simulink model "STEMMS_VOLTAGE_COMMENTED_V2"  (R2019b)
settings: Solver=FixedStepAuto  StartTime=0.0  StopTime=inf  RelTol=1e-3
libraries: vexarmcortexlib x26, vexcommonlib x7
settings Model: ExtModeTrigDuration=25  Creator=nicoa  LastModifiedBy=nicoa
settings OptimizationCC: EnhancedBackFolding=on  PassReuseOutputArgsAs=Individual arguments  ZeroExternalMemoryAtStartup=off  ZeroInternalMemoryAtStartup=off  MaxStackSize=64  OptimizeBlockOrder=speed  DifferentSizesBufferReuse=on  OptimizationCustomize=off  EfficientTunableParamExpr=on
settings DebuggingCC: ParameterTunabilityLossMsg=error
settings HardwareCC: ProdBitPerPointer=32  ProdBitPerSizeT=32  ProdBitPerPtrDiffT=32  ProdLargestAtomicInteger=Long  ProdLargestAtomicFloat=Double  ProdWordSize=32  ProdHWDeviceType=ARM Compatible->ARM Cortex
settings SFSimCC: MATLABDynamicMemAlloc=off
settings RTWCC: SystemTargetFile=ert.tlc  HardwareBoard=ARM Cortex-based VEX Microcontroller  TLCOptions="-aInlineSetEventsForThisBaseRateFcn=TLC_FALSE -aSuppressMultiTaskScheduler=TLC_FALSE  -aRateBasedStepFcn=0"  TemplateMakefile=ert_default_tmf  GenerateReport=on  Toolchain=GNU Tools for VEX ARM Cortex  IncludeHyperlinkInReport=on  LaunchReport=on  GenerateTraceInfo=on  GenerateTraceReport=on  GenerateTraceReportSl=on  GenerateTraceReportSf=on  GenerateTraceReportEml=on
settings CodeAppCC: ForceParamTrailComments=on  IgnoreCustomStorageClasses=off  OperatorAnnotations=on  SimulinkDataObjDesc=on  SFDataObjDesc=on  InsertBlockDesc=on

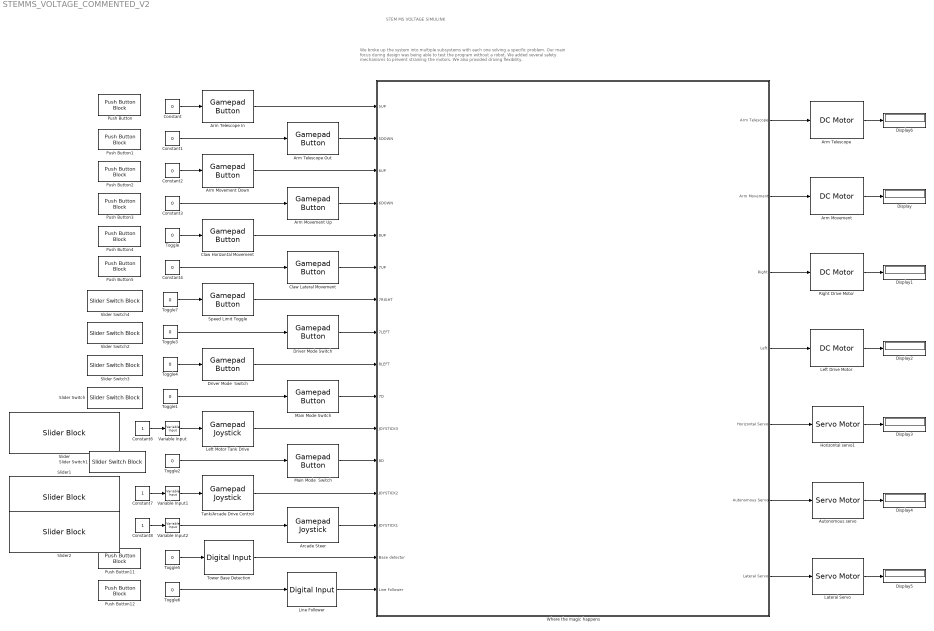
== system STEMMS_VOLTAGE_COMMENTED_V2 ==
  note: We broke up the system into multiple subsystems with each one solving a specific problem. Our main focus during
      | design was being able to test the program without a robot. We added several safety mechanisms to prevent straining
      |  the motors. We also provided driving flexibility.
  note: STEM MS VOLTAGE SIMULINK
  "Arcade Steer " : vexarmcortexlib/Gamepad/Gamepad Joystick  joystick=1  chan=1  SimulationIn=on  SampleTime=0.02
      settings: SourceProductName=Simulink Coder Support Package for ARM Cortex-based VEX Microcontroller  SourceProductBaseCode=EC_VEX_MICRO
  Arm Movement : vexarmcortexlib/Actuators/DC Motor  motor=6  scaleFactor=1/13.5  SimulationOut=on
      settings: SourceProductName=Simulink Coder Support Package for ARM Cortex-based VEX Microcontroller  SourceProductBaseCode=EC_VEX_MICRO
  Arm Movement Down : vexarmcortexlib/Gamepad/Gamepad Button  joystick=1  chan=6  button56=Down  button78=Down  SimulationIn=on  SampleTime=0.02
      settings: SourceProductName=Simulink Coder Support Package for ARM Cortex-based VEX Microcontroller  SourceProductBaseCode=EC_VEX_MICRO
  Arm Movement Up : vexarmcortexlib/Gamepad/Gamepad Button  joystick=1  chan=6  button56=Up  button78=Down  SimulationIn=on  SampleTime=0.02
      settings: SourceProductName=Simulink Coder Support Package for ARM Cortex-based VEX Microcontroller  SourceProductBaseCode=EC_VEX_MICRO
  Arm Telescope : vexarmcortexlib/Actuators/DC Motor  motor=2  scaleFactor=1/13.5  SimulationOut=on
      settings: SourceProductName=Simulink Coder Support Package for ARM Cortex-based VEX Microcontroller  SourceProductBaseCode=EC_VEX_MICRO
  Arm Telescope In : vexarmcortexlib/Gamepad/Gamepad Button  joystick=1  chan=5  button56=Down  button78=Down  SimulationIn=on  SampleTime=0.02
      settings: SourceProductName=Simulink Coder Support Package for ARM Cortex-based VEX Microcontroller  SourceProductBaseCode=EC_VEX_MICRO
  Arm Telescope Out : vexarmcortexlib/Gamepad/Gamepad Button  joystick=1  chan=5  button56=Up  button78=Down  SimulationIn=on  SampleTime=0.02
      settings: SourceProductName=Simulink Coder Support Package for ARM Cortex-based VEX Microcontroller  SourceProductBaseCode=EC_VEX_MICRO
  Autonomous servo : vexarmcortexlib/Actuators/Servo Motor  motor=5  scaleFactor=60/127  SimulationOut=on
      settings: SourceProductName=Simulink Coder Support Package for ARM Cortex-based VEX Microcontroller  SourceProductBaseCode=EC_VEX_MICRO
  Claw Horizontal Movement : vexarmcortexlib/Gamepad/Gamepad Button  joystick=1  chan=8  button56=Up  button78=Up  SimulationIn=on  SampleTime=0.02
      settings: SourceProductName=Simulink Coder Support Package for ARM Cortex-based VEX Microcontroller  SourceProductBaseCode=EC_VEX_MICRO
  Claw Lateral Movement : vexarmcortexlib/Gamepad/Gamepad Button  joystick=1  chan=7  button56=Up  button78=Up  SimulationIn=on  SampleTime=0.02
      settings: SourceProductName=Simulink Coder Support Package for ARM Cortex-based VEX Microcontroller  SourceProductBaseCode=EC_VEX_MICRO
  Constant{,1..4} (5 alike) : Constant  Value=0
  Constant6 : Constant
  Constant7 : Constant
  Constant8 : Constant
  Display{,1..6} (7 alike) : Display
  Driver Mode  Switch : vexarmcortexlib/Gamepad/Gamepad Button  joystick=1  chan=8  button56=Up  button78=Left  SimulationIn=on  SampleTime=0.02
      settings: SourceProductName=Simulink Coder Support Package for ARM Cortex-based VEX Microcontroller  SourceProductBaseCode=EC_VEX_MICRO
  Driver Mode Switch : vexarmcortexlib/Gamepad/Gamepad Button  joystick=1  chan=7  button56=Up  button78=Left  SimulationIn=on  SampleTime=0.02
      settings: SourceProductName=Simulink Coder Support Package for ARM Cortex-based VEX Microcontroller  SourceProductBaseCode=EC_VEX_MICRO
  Horizontal servo1 : vexarmcortexlib/Actuators/Servo Motor  motor=7  scaleFactor=60/127  SimulationOut=on
      settings: SourceProductName=Simulink Coder Support Package for ARM Cortex-based VEX Microcontroller  SourceProductBaseCode=EC_VEX_MICRO
  Lateral Servo : vexarmcortexlib/Actuators/Servo Motor  motor=3  scaleFactor=60/127  SimulationOut=on
      settings: SourceProductName=Simulink Coder Support Package for ARM Cortex-based VEX Microcontroller  SourceProductBaseCode=EC_VEX_MICRO
  "Left Drive Motor " : vexarmcortexlib/Actuators/DC Motor  motor=9  scaleFactor=1/13.5  SimulationOut=on
      settings: SourceProductName=Simulink Coder Support Package for ARM Cortex-based VEX Microcontroller  SourceProductBaseCode=EC_VEX_MICRO
  Left Motor Tank Drive : vexarmcortexlib/Gamepad/Gamepad Joystick  joystick=1  chan=3  SimulationIn=on  SampleTime=0.02
      settings: SourceProductName=Simulink Coder Support Package for ARM Cortex-based VEX Microcontroller  SourceProductBaseCode=EC_VEX_MICRO
  Line Follower : vexarmcortexlib/Sensors/Digital Input  inChan=1  SimulationIn=on  SampleTime=0.2
      settings: SourceProductName=Simulink Coder Support Package for ARM Cortex-based VEX Microcontroller  SourceProductBaseCode=EC_VEX_MICRO
  Main Mode  Switch : vexarmcortexlib/Gamepad/Gamepad Button  joystick=1  chan=8  button56=Up  button78=Down  SimulationIn=on  SampleTime=0.02
      settings: SourceProductName=Simulink Coder Support Package for ARM Cortex-based VEX Microcontroller  SourceProductBaseCode=EC_VEX_MICRO
  Main Mode Switch : vexarmcortexlib/Gamepad/Gamepad Button  joystick=1  chan=7  button56=Up  button78=Down  SimulationIn=on  SampleTime=0.02
      settings: SourceProductName=Simulink Coder Support Package for ARM Cortex-based VEX Microcontroller  SourceProductBaseCode=EC_VEX_MICRO
  Push Button{,1..5,11..12} (8 alike) : PushButtonBlock
  Right Drive Motor : vexarmcortexlib/Actuators/DC Motor  motor=4  scaleFactor=1/13.5  SimulationOut=on
      settings: SourceProductName=Simulink Coder Support Package for ARM Cortex-based VEX Microcontroller  SourceProductBaseCode=EC_VEX_MICRO
  Slider : SliderBlock  LabelPosition=Hide  ScaleMin=-127  ScaleMax=127
  Slider Switch{,1..4} (5 alike) : SliderSwitchBlock  LabelPosition=Hide
      settings: Values={{'Off', 'On'}, [0 1]}
  Slider1 : SliderBlock  LabelPosition=Hide  ScaleMin=-127  ScaleMax=127
  Slider2 : SliderBlock  LabelPosition=Hide  ScaleMin=-127  ScaleMax=127
  Speed Limit Toggle : vexarmcortexlib/Gamepad/Gamepad Button  joystick=1  chan=7  button56=Up  button78=Right  SimulationIn=on  SampleTime=0.02
      settings: SourceProductName=Simulink Coder Support Package for ARM Cortex-based VEX Microcontroller  SourceProductBaseCode=EC_VEX_MICRO
  Tank/Arcade Drive Control : vexarmcortexlib/Gamepad/Gamepad Joystick  joystick=1  chan=2  SimulationIn=on  SampleTime=0.02
      settings: SourceProductName=Simulink Coder Support Package for ARM Cortex-based VEX Microcontroller  SourceProductBaseCode=EC_VEX_MICRO
  Toggle{,1..7} (8 alike) : Constant  Value=0
      settings: OpenFcn=|
      | if strcmp('0',get_param(gcb, 'Value'))                        set_param(gcb, 'Value', '1');
      | else
      |             set_param(gcb, 'Value', '0');
      | end
  Tower Base Detection : vexarmcortexlib/Sensors/Digital Input  inChan=11  SimulationIn=on  SampleTime=0.2
      settings: SourceProductName=Simulink Coder Support Package for ARM Cortex-based VEX Microcontroller  SourceProductBaseCode=EC_VEX_MICRO
  Variable Input : vexarmcortexlib/Utilities/Variable Input  low=-127  gain=94.76544331395348  high=127
      settings: SourceProductName=Simulink Coder Support Package for ARM Cortex-based VEX Microcontroller  SourceProductBaseCode=EC_VEX_MICRO
  Variable Input1 : vexarmcortexlib/Utilities/Variable Input  low=-127  gain=-87  high=127
      settings: SourceProductName=Simulink Coder Support Package for ARM Cortex-based VEX Microcontroller  SourceProductBaseCode=EC_VEX_MICRO
  Variable Input2 : vexarmcortexlib/Utilities/Variable Input  low=-127  gain=56.37009447674421  high=127
      settings: SourceProductName=Simulink Coder Support Package for ARM Cortex-based VEX Microcontroller  SourceProductBaseCode=EC_VEX_MICRO
  Where the magic happens : Subsystem
  wires:
  Main Mode  Switch/1 -> Where the magic happens/12(8D)
  Main Mode Switch/1 -> Where the magic happens/10(7D)
  Where the magic happens/4(Left) -> "Left Drive Motor "/1
  Where the magic happens/6(Autonomous Servo) -> Autonomous servo/1
  Tower Base Detection/1 -> Where the magic happens/15(Base detector)
  Line Follower/1 -> Where the magic happens/16(Line Follower)
  Driver Mode  Switch/1 -> Where the magic happens/9(8LEFT)
  Driver Mode Switch/1 -> Where the magic happens/8(7LEFT)
  Speed Limit Toggle/1 -> Where the magic happens/7(7RIGHT)
  Tank/Arcade Drive Control/1 -> Where the magic happens/13(JOYSTICK2)
  Left Motor Tank Drive/1 -> Where the magic happens/11(JOYSTICK3)
  "Arcade Steer "/1 -> Where the magic happens/14(JOYSTICK1)
  Where the magic happens/3(Right) -> Right Drive Motor/1
  Where the magic happens/7(Lateral Servo) -> Lateral Servo/1
  Where the magic happens/5(Horizontal Servo) -> Horizontal servo1/1
  Claw Lateral Movement/1 -> Where the magic happens/6(7UP)
  Claw Horizontal Movement/1 -> Where the magic happens/5(8UP)
  Where the magic happens/2(Arm Movement) -> Arm Movement/1
  Arm Movement Up/1 -> Where the magic happens/4(6DOWN)
  Arm Movement Down/1 -> Where the magic happens/3(6UP)
  Where the magic happens/1(Arm Telescope) -> Arm Telescope/1
  Arm Telescope Out/1 -> Where the magic happens/2(5DOWN)
  Arm Telescope In/1 -> Where the magic happens/1(5UP)
  Arm Movement/1 -> Display/1
  Right Drive Motor/1 -> Display1/1
  "Left Drive Motor "/1 -> Display2/1
  Horizontal servo1/1 -> Display3/1
  Autonomous servo/1 -> Display4/1
  Lateral Servo/1 -> Display5/1
  Arm Telescope/1 -> Display6/1
  Constant/1 -> Arm Telescope In/1
  Constant1/1 -> Arm Telescope Out/1
  Constant2/1 -> Arm Movement Down/1
  Constant3/1 -> Arm Movement Up/1
  Toggle/1 -> Claw Horizontal Movement/1
  Constant4/1 -> Claw Lateral Movement/1
  Toggle7/1 -> Speed Limit Toggle/1
  Toggle4/1 -> Driver Mode  Switch/1
  Toggle1/1 -> Main Mode Switch/1
  Constant6/1 -> Variable Input/1
  Variable Input/1 -> Left Motor Tank Drive/1
  Variable Input1/1 -> Tank/Arcade Drive Control/1
  Constant7/1 -> Variable Input1/1
  Variable Input2/1 -> "Arcade Steer "/1
  Constant8/1 -> Variable Input2/1
  Toggle2/1 -> Main Mode  Switch/1
  Toggle5/1 -> Tower Base Detection/1
  Toggle6/1 -> Line Follower/1
  Toggle3/1 -> Driver Mode Switch/1

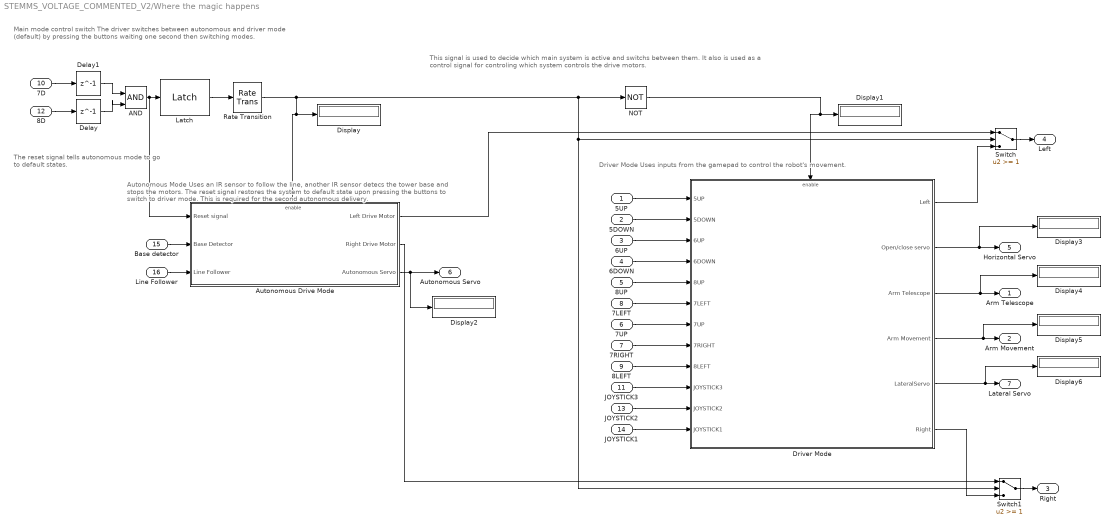
== system STEMMS_VOLTAGE_COMMENTED_V2/Where the magic happens ==
  note: Driver Mode
      | Uses inputs from the gamepad to control the robot's movement.
  note: This signal is used to decide which main system is active and switchs between them.
      | It also is used as a control signal for controling which system controls the drive motors.
  note: The reset signal tells autonomous
      | mode to go to default states.
  note: Autonomous Mode
      | Uses an IR sensor to follow the line, another IR sensor detecs the
      | tower base and stops the motors. The reset signal restores the system
      | to default state upon pressing the buttons to switch to driver mode. This
      | is required for the second autonomous delivery.
  note: Main mode control switch
      | The driver switches between autonomous and driver mode (default) by
      | pressing the buttons waiting one second then switching modes.
  5UP : Inport
  5DOWN : Inport  Port=2
  6UP : Inport  Port=3
  6DOWN : Inport  Port=4
  8UP : Inport  Port=5
  7UP : Inport  Port=6
  7RIGHT : Inport  Port=7
  7LEFT : Inport  Port=8
  8LEFT : Inport  Port=9
  7D : Inport  Port=10
  JOYSTICK3 : Inport  Port=11
  8D : Inport  Port=12
  JOYSTICK2 : Inport  Port=13
  JOYSTICK1 : Inport  Port=14
  Base detector : Inport  Port=15
  Line Follower : Inport  Port=16
  "AND " : Logic  IconShape=distinctive  AllPortsSameDT=off  OutDataTypeStr=boolean
  Autonomous Drive Mode : Subsystem
  Delay : Delay  DelayLength=1  InitialCondition=0  SampleTime=1
  Delay1 : Delay  DelayLength=1  InitialCondition=0  SampleTime=1
  Display{,1..6} (7 alike) : Display
  Driver Mode : Subsystem  TreatAsAtomicUnit=on
  Latch : vexcommonlib/Latch  output0=off  BlockPlatform=vexarmcortex
      settings: SourceProductName=Simulink Coder Support Package for ARM Cortex-based VEX Microcontroller  SourceProductBaseCode=EC_VEX_MICRO
  NOT : Logic  Operator=NOT  IconShape=distinctive  AllPortsSameDT=off  OutDataTypeStr=boolean
  Rate Transition : RateTransition
  Switch : Switch  Threshold=1
  Switch1 : Switch  Threshold=1
  Arm Telescope : Outport
  Arm Movement : Outport  Port=2
  Right : Outport  Port=3
  Left : Outport  Port=4
  Horizontal Servo : Outport  Port=5
  Autonomous Servo : Outport  Port=6
  Lateral Servo : Outport  Port=7
  wires:
  "AND "/1 -> Autonomous Drive Mode/1(Reset signal), Latch/1
  Delay1/1 -> "AND "/1
  Latch/1 -> Rate Transition/1
  7D/1 -> Delay1/1
  Delay/1 -> "AND "/2
  8D/1 -> Delay/1
  Autonomous Drive Mode/3(Autonomous Servo) -> Display2/1, Autonomous Servo/1
  Rate Transition/1 -> Display/1, Autonomous Drive Mode/Enable, NOT/1, Switch1/2, Switch/2
  NOT/1 -> Display1/1, Driver Mode/Enable
  Autonomous Drive Mode/1(Left Drive Motor) -> Switch/1
  Switch/1 -> Left/1
  Autonomous Drive Mode/2(Right Drive Motor) -> Switch1/1
  Switch1/1 -> Right/1
  Line Follower/1 -> Autonomous Drive Mode/3(Line Follower)
  Base detector/1 -> Autonomous Drive Mode/2(Base Detector)
  7RIGHT/1 -> Driver Mode/8(7RIGHT)
  JOYSTICK3/1 -> Driver Mode/10(JOYSTICK3)
  JOYSTICK2/1 -> Driver Mode/11(JOYSTICK2)
  JOYSTICK1/1 -> Driver Mode/12(JOYSTICK1)
  Driver Mode/5(LateralServo) -> Display6/1, Lateral Servo/1
  Driver Mode/2(Open/close servo) -> Display3/1, Horizontal Servo/1
  8UP/1 -> Driver Mode/5(8UP)
  7UP/1 -> Driver Mode/7(7UP)
  Driver Mode/4(Arm Movement) -> Display5/1, Arm Movement/1
  Driver Mode/3(Arm Telescope) -> Display4/1, Arm Telescope/1
  Driver Mode/6(Right) -> Switch1/3
  Driver Mode/1(Left) -> Switch/3
  5DOWN/1 -> Driver Mode/2(5DOWN)
  5UP/1 -> Driver Mode/1(5UP)
  6UP/1 -> Driver Mode/3(6UP)
  6DOWN/1 -> Driver Mode/4(6DOWN)
  7LEFT/1 -> Driver Mode/6(7LEFT)
  8LEFT/1 -> Driver Mode/9(8LEFT)

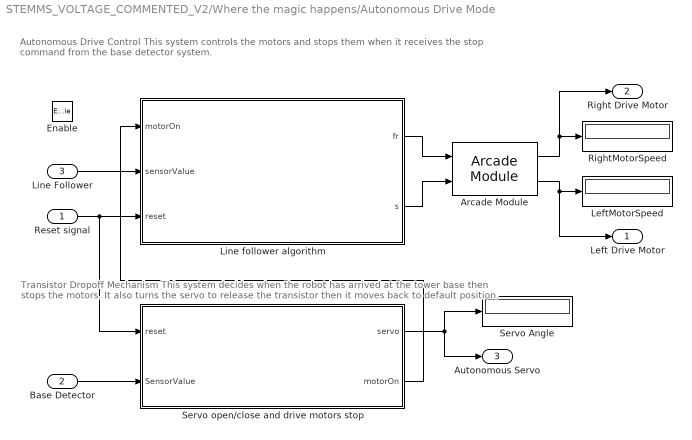
== system STEMMS_VOLTAGE_COMMENTED_V2/Where the magic happens/Autonomous Drive Mode ==
  note: Transistor Dropoff Mechanism
      | This system decides when the robot has arrived at the tower base then stops the motors. It also turns the servo to
      | release the transistor then it moves back to default position.
  note: Autonomous Drive Control
      | This system controls the motors and stops them when it receives the stop command from the base detector system.
  Reset signal : Inport
  Base Detector : Inport  Port=2
  Line Follower : Inport  Port=3
  Enable : EnablePort
  Arcade Module : vexcommonlib/Arcade Module  BlockPlatform=vexarmcortex
      settings: SourceProductName=Simulink Coder Support Package for ARM Cortex-based VEX Microcontroller  SourceProductBaseCode=EC_VEX_MICRO
  LeftMotorSpeed : Display
  Line follower algorithm : Stateflow chart  TreatAsAtomicUnit=on
  RightMotorSpeed : Display
  Servo Angle : Display
  Servo open/close and drive motors stop : Stateflow chart  TreatAsAtomicUnit=on
  Left Drive Motor : Outport
  Right Drive Motor : Outport  Port=2
  Autonomous Servo : Outport  Port=3
  wires:
  Base Detector/1 -> Servo open/close and drive motors stop/2(SensorValue)
  Line Follower/1 -> Line follower algorithm/2(sensorValue)
  Line follower algorithm/2(s) -> Arcade Module/2
  Line follower algorithm/1(fr) -> Arcade Module/1
  Arcade Module/1 -> RightMotorSpeed/1, Right Drive Motor/1
  Arcade Module/2 -> LeftMotorSpeed/1, Left Drive Motor/1
  Servo open/close and drive motors stop/1(servo) -> Autonomous Servo/1, Servo Angle/1
  Servo open/close and drive motors stop/2(motorOn) -> Line follower algorithm/1(motorOn)
  Reset signal/1 -> Servo open/close and drive motors stop/1(reset), Line follower algorithm/3(reset)

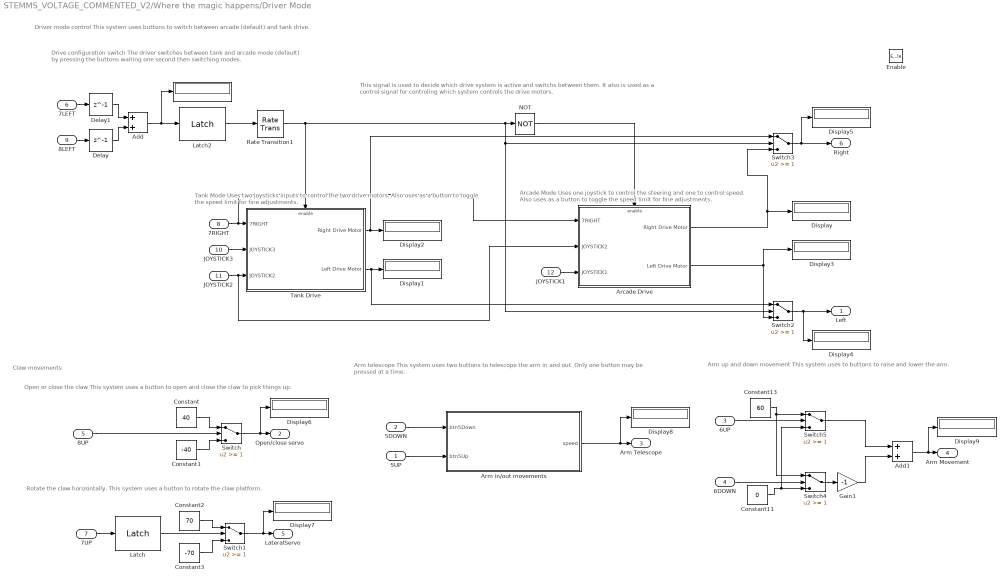
== system STEMMS_VOLTAGE_COMMENTED_V2/Where the magic happens/Driver Mode ==
  note: Rotate the claw horizontally.
      | This system uses a button to rotate the claw platform.
  note: Open or close the claw
      | This system uses a button to open and close the
      | claw to pick things up.
  note: Arcade Mode
      | Uses one joystick to control the steering and one to control
      | speed. Also uses as a button to toggle the speed limit for fine
      | adjustments.
  note: Tank Mode
      | Uses two joysticks inputs to control the two drive motors. Also uses as a button
      | to toggle the speed limit for fine adjustments.
  note: Drive configuration switch
      | The driver switches between tank and arcade mode (default) by
      | pressing the buttons waiting one second then switching modes.
  note: Arm telescope
      | This system uses two buttons to telescope the arm in and out.
      | Only one button may be pressed at a time.
  note: Claw movements
  note: Arm up and down movement
      | This system uses to buttons to raise and lower the arm.
  note: Driver mode control
      | This system uses buttons to switch between arcade (default) and tank drive.
  note: This signal is used to decide which drive system is active and switchs between them.
      | It also is used as a control signal for controling which system controls the drive motors.
  5UP : Inport
  5DOWN : Inport  Port=2
  6UP : Inport  Port=3
  6DOWN : Inport  Port=4
  8UP : Inport  Port=5
  7LEFT : Inport  Port=6
  7UP : Inport  Port=7
  7RIGHT : Inport  Port=8
  8LEFT : Inport  Port=9
  JOYSTICK3 : Inport  Port=10
  JOYSTICK2 : Inport  Port=11
  JOYSTICK1 : Inport  Port=12
  Enable : EnablePort
  " " : Display
  Add : Sum
  Add1 : Sum
  "Arcade Drive " : Subsystem  TreatAsAtomicUnit=on
  Arm in/out movements : Stateflow chart  BlockKeywords=__PRM__SERIALIZED__DATA__:Stateflow Chart,Stateflow Diagram  TreatAsAtomicUnit=on
  Constant : Constant  Value=40
  Constant1 : Constant  Value=-40
  Constant11 : Constant  Value=0
  Constant13 : Constant  Value=60
  Constant2 : Constant  Value=70
  Constant3 : Constant  Value=-70
  Delay : Delay  DelayLength=1  InitialCondition=0  SampleTime=1
  Delay1 : Delay  DelayLength=1  InitialCondition=0  SampleTime=1
  Display{,1..9} (10 alike) : Display
  Gain1 : Gain  Gain=-1
  Latch : vexcommonlib/Latch  output0=off  BlockPlatform=vexarmcortex
      settings: SourceProductName=Simulink Coder Support Package for ARM Cortex-based VEX Microcontroller  SourceProductBaseCode=EC_VEX_MICRO
  Latch2 : vexcommonlib/Latch  output0=off  BlockPlatform=vexarmcortex
      settings: SourceProductName=Simulink Coder Support Package for ARM Cortex-based VEX Microcontroller  SourceProductBaseCode=EC_VEX_MICRO
  NOT : Logic  Operator=NOT  IconShape=distinctive  AllPortsSameDT=off  OutDataTypeStr=boolean
  Rate Transition1 : RateTransition
  Switch{,1..5} (6 alike) : Switch  Threshold=1
  "Tank Drive " : Subsystem  TreatAsAtomicUnit=on
  Left : Outport
  Open/close servo : Outport  Port=2
  Arm Telescope : Outport  Port=3
  Arm Movement : Outport  Port=4
  LateralServo : Outport  Port=5
  Right : Outport  Port=6
  wires:
  Rate Transition1/1 -> NOT/1, Switch2/2, Switch3/2, "Tank Drive "/Enable
  7LEFT/1 -> Delay1/1
  NOT/1 -> "Arcade Drive "/Enable
  Delay1/1 -> Add/1
  Delay/1 -> Add/2
  Latch2/1 -> Rate Transition1/1
  Add/1 -> " "/1, Latch2/1
  8LEFT/1 -> Delay/1
  JOYSTICK3/1 -> "Tank Drive "/2(JOYSTICK3)
  JOYSTICK2/1 -> "Tank Drive "/3(JOYSTICK2), "Arcade Drive "/2(JOYSTICK2)
  JOYSTICK1/1 -> "Arcade Drive "/3(JOYSTICK1)
  Constant/1 -> Switch/1
  7UP/1 -> Latch/1
  Latch/1 -> Switch1/2
  Switch/1 -> Display6/1, Open/close servo/1
  Constant1/1 -> Switch/3
  Switch1/1 -> Display7/1, LateralServo/1
  Constant2/1 -> Switch1/1
  Constant3/1 -> Switch1/3
  Switch4/1 -> Gain1/1
  Constant11/1 -> Switch5/3, Switch4/3
  6DOWN/1 -> Switch4/2
  6UP/1 -> Switch5/2
  Constant13/1 -> Switch5/1, Switch4/1
  Add1/1 -> Display9/1, Arm Movement/1
  5UP/1 -> Arm in/out movements/2(btn5Up)
  Arm in/out movements/1(speed) -> Display8/1, Arm Telescope/1
  5DOWN/1 -> Arm in/out movements/1(btn5Down)
  Switch2/1 -> Display4/1, Left/1
  "Arcade Drive "/2(Left Drive Motor) -> Switch2/3, Display3/1
  Switch3/1 -> Display5/1, Right/1
  "Arcade Drive "/1(Right Drive Motor) -> Display/1, Switch3/3
  7RIGHT/1 -> "Tank Drive "/1(7RIGHT), "Arcade Drive "/1(7RIGHT)
  "Tank Drive "/2(Left Drive Motor) -> Display1/1, Switch2/1
  "Tank Drive "/1(Right Drive Motor) -> Display2/1, Switch3/1
  Switch5/1 -> Add1/1
  Gain1/1 -> Add1/2
  8UP/1 -> Switch/2

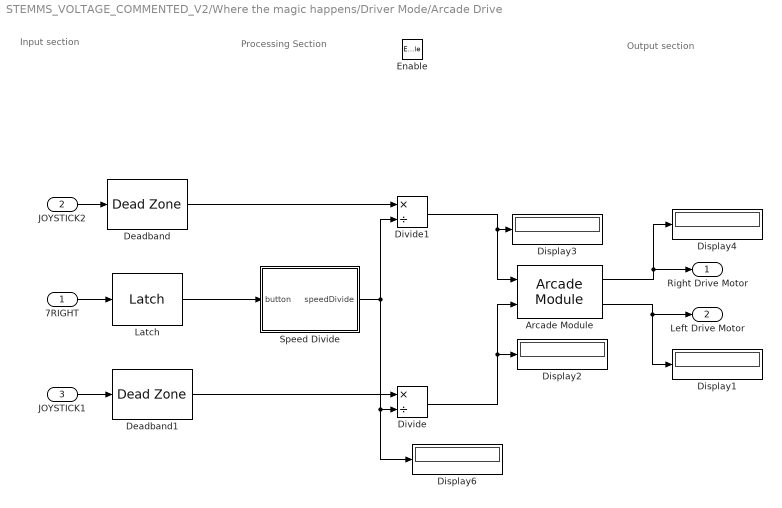
== system STEMMS_VOLTAGE_COMMENTED_V2/Where the magic happens/Driver Mode/Arcade Drive  ==
  note: Output section
  note: Processing Section
  note: Input section
  7RIGHT : Inport
  JOYSTICK2 : Inport  Port=2
  JOYSTICK1 : Inport  Port=3
  Enable : EnablePort
  Arcade Module : vexcommonlib/Arcade Module  BlockPlatform=vexarmcortex
      settings: SourceProductName=Simulink Coder Support Package for ARM Cortex-based VEX Microcontroller  SourceProductBaseCode=EC_VEX_MICRO
  Deadband : DeadZone  LowerValue=-5  UpperValue=5  SaturateOnIntegerOverflow=on
  Deadband1 : DeadZone  LowerValue=-5  UpperValue=5  SaturateOnIntegerOverflow=on
  Display{1..4,6} (5 alike) : Display
  Divide : Product  Inputs=*/
  Divide1 : Product  Inputs=*/
  Latch : vexcommonlib/Latch  output0=off  BlockPlatform=vexarmcortex
      settings: SourceProductName=Simulink Coder Support Package for ARM Cortex-based VEX Microcontroller  SourceProductBaseCode=EC_VEX_MICRO
  Speed Divide : Stateflow chart  TreatAsAtomicUnit=on
  Right Drive Motor : Outport
  Left Drive Motor : Outport  Port=2
  wires:
  JOYSTICK1/1 -> Deadband1/1
  JOYSTICK2/1 -> Deadband/1
  7RIGHT/1 -> Latch/1
  Speed Divide/1(speedDivide) -> Display6/1, Divide/2, Divide1/2
  Deadband/1 -> Divide1/1
  Deadband1/1 -> Divide/1
  Divide/1 -> Arcade Module/2, Display2/1
  Divide1/1 -> Arcade Module/1, Display3/1
  Arcade Module/1 -> Display4/1, Right Drive Motor/1
  Arcade Module/2 -> Display1/1, Left Drive Motor/1
  Latch/1 -> Speed Divide/1(button)

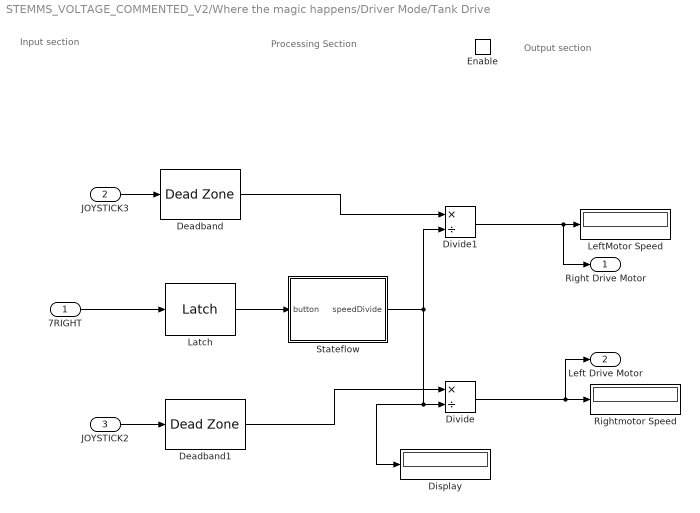
== system STEMMS_VOLTAGE_COMMENTED_V2/Where the magic happens/Driver Mode/Tank Drive  ==
  note: Output section
  note: Processing Section
  note: Input section
  7RIGHT : Inport
  JOYSTICK3 : Inport  Port=2
  JOYSTICK2 : Inport  Port=3
  Enable : EnablePort
  Deadband : DeadZone  LowerValue=-5  UpperValue=5  SaturateOnIntegerOverflow=on
  Deadband1 : DeadZone  LowerValue=-5  UpperValue=5  SaturateOnIntegerOverflow=on
  Display : Display
  Divide : Product  Inputs=*/
  Divide1 : Product  Inputs=*/
  Latch : vexcommonlib/Latch  output0=off  BlockPlatform=vexarmcortex
      settings: SourceProductName=Simulink Coder Support Package for ARM Cortex-based VEX Microcontroller  SourceProductBaseCode=EC_VEX_MICRO
  LeftMotor Speed : Display
  Rightmotor Speed : Display
  Stateflow : Stateflow chart  TreatAsAtomicUnit=on
  Right Drive Motor : Outport
  Left Drive Motor : Outport  Port=2
  wires:
  JOYSTICK3/1 -> Deadband/1
  7RIGHT/1 -> Latch/1
  Latch/1 -> Stateflow/1(button)
  Stateflow/1(speedDivide) -> Divide1/2, Display/1, Divide/2
  Deadband/1 -> Divide1/1
  Divide1/1 -> Right Drive Motor/1, LeftMotor Speed/1
  JOYSTICK2/1 -> Deadband1/1
  Divide/1 -> Left Drive Motor/1, Rightmotor Speed/1
  Deadband1/1 -> Divide/1

== stateflow chart STEMMS_VOLTAGE_COMMENTED_V2/Where the magic happens/Autonomous Drive Mode/Line follower algorithm ==
  state GO_RIGHT
    entry:
    fr = 50;
    s = -50;
  state GO_LEFT
    entry:
    fr = 50;
    s = 50;
  state STOPPED
    entry:
    fr = 0;
    s = 0;
  (default) -> GO_LEFT
  GO_LEFT -> GO_RIGHT [order 2] : [sensorValue == 1]
  GO_RIGHT -> GO_LEFT [order 2] : [sensorValue == 0]
  STOPPED -> GO_LEFT [order 2] : [sensorValue == 0 && reset == 0]
  GO_LEFT -> STOPPED [order 1] : [motorOn == 0]
  GO_RIGHT -> STOPPED [order 1] : [motorOn == 0]
  STOPPED -> GO_RIGHT [order 1] : [sensorValue == 1 && reset == 0]
  data: fr output; s output; motorOn input; sensorValue input; reset input

== stateflow chart STEMMS_VOLTAGE_COMMENTED_V2/Where the magic happens/Driver Mode/Arcade Drive /Speed Divide ==
  state Full_Speed
    entry:
    speedDivide = 1
  state Slow_Speed
    entry:
    speedDivide = 4
  (default) -> Full_Speed
  Full_Speed -> Slow_Speed : [button == 1]
  Slow_Speed -> Full_Speed : [button == 0]
  data: speedDivide output; button input

== stateflow chart STEMMS_VOLTAGE_COMMENTED_V2/Where the magic happens/Driver Mode/Tank Drive /Stateflow ==
  state Full_Speed
    entry:
    speedDivide = 1
  state Slow_Speed
    entry:
    speedDivide = 4
  (default) -> Full_Speed
  Full_Speed -> Slow_Speed : [button]
  Slow_Speed -> Full_Speed : [button == 0]
  data: speedDivide output; button input

== stateflow chart STEMMS_VOLTAGE_COMMENTED_V2/Where the magic happens/Autonomous Drive Mode/Servo open//close and drive motors stop ==
  state move
    entry:
    servo = 0;
    motorOn = 1;
  state Stop
    entry:
    servo = 67;
    motorOn = 0;
  state off
    entry:
    servo = 0;
    motorOn = 0;
  (default) -> move
  off -> move : [reset == 0]
  move -> Stop : [SensorValue == 1]
  Stop -> off : [after(3,sec)]
  data: reset input; SensorValue input; servo output; motorOn output

== stateflow chart STEMMS_VOLTAGE_COMMENTED_V2/Where the magic happens/Driver Mode/Arm in//out movements ==
  state ARMDOWN
    entry:
    speed = -40;
  state STOPPED
    entry:
    speed = 0;
  state ARMUP
    entry:
    speed = 40;
  (default) -> STOPPED
  STOPPED -> ARMUP [order 1] : [btn5Down == 0 && btn5Up == 1 ]
  STOPPED -> ARMDOWN [order 2] : [btn5Down == 1 && btn5Up == 0]
  ARMDOWN -> STOPPED [order 2] : [btn5Down == 0]
  ARMUP -> STOPPED [order 2] : [btn5Up == 0]
  ARMDOWN -> STOPPED [order 1] : [btn5Down == 1 && btn5Up == 1]
  ARMUP -> STOPPED [order 1] : [btn5Down == 1 && btn5Up == 1]
  data: btn5Down input; btn5Up input; speed output
